simulink model "plt_aut_full"  (R2014a)
settings: Solver=ode45  StartTime=0.0  StopTime=70  MaxStep=0.01  RelTol=1e-3
values from neighbouring files (symbols this model uses):
  alpha = 1+1/(k*beta)    (= 1.025)    [tp1_syst_asservis.m]
  beta = 4    [tp1_syst_asservis.m]
  k = 10    [tp1_syst_asservis.m]
  Kd = 0.0001    [tp1_syst_asservis.m]
  Te = 0.2    [tp1_syst_asservis.m]
  to = 1.2    [tp1_syst_asservis.m]
settings Model: Creator=12210406  LastModifiedBy=UTILISATEUR
settings OptimizationCC: BlockReduction=off  BooleanDataType=off  SimCompilerOptimization=off
settings DebuggingCC: SaveWithParameterizedLinksMsg=none  UnderspecifiedInitializationDetection=Classic  SignalResolutionControl=TryResolveAllWithWarning  SolverPrmCheckMsg=none  FcnCallInpInsideContextMsg=error  FrameProcessingCompatibilityMsg=error  LibraryContextMissingDiagnostic=warning  SFExecutionAtInitializationDiag=none
settings HardwareCC: ProdBitPerSizeT=32  ProdBitPerPtrDiffT=32  TargetUnknown=on
settings RTWCC: RTWCompilerOptimization=off
settings CodeAppCC: StateflowObjectComments=on
settings ConfigComp: CovMetricSettings=dw  CovHtmlReporting=on  CovSaveCumulativeToWorkspaceVar=on  CovSaveSingleToWorkspaceVar=on  CovExternalEMLEnable=off  CovSFcnEnable=off

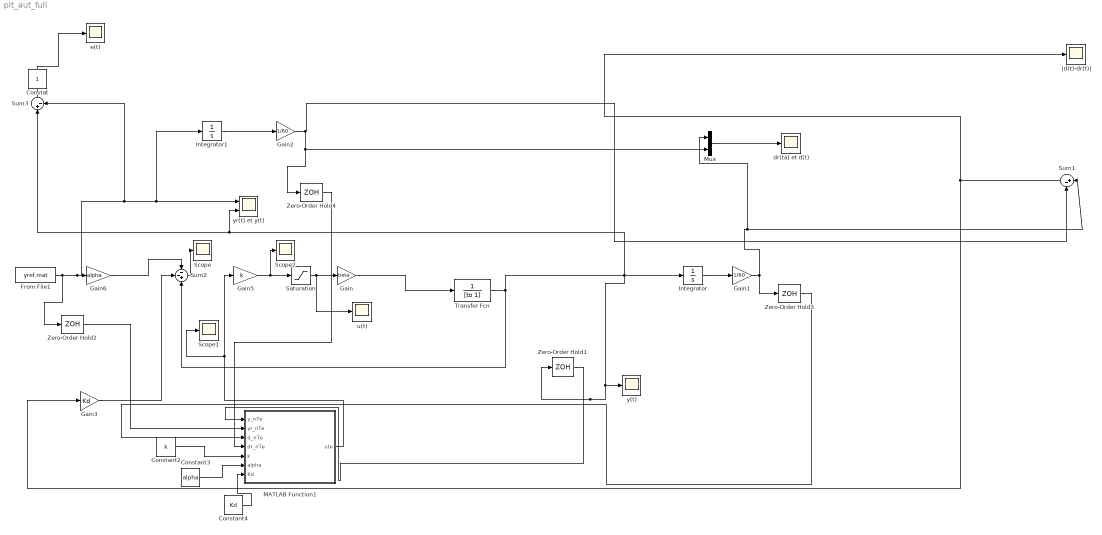
== system plt_aut_full ==
  Constant2 : Constant  Value=k
  Constant3 : Constant  Value=alpha
  Constant4 : Constant  Value=Kd
  From File1 : FromFile  FileName=yref.mat  SampleTime=0
  Gain : Gain  Gain=beta
  Gain1 : Gain  Gain=1/60
  Gain2 : Gain  Gain=1/60
  Gain3 : Gain  Gain=Kd
  Gain5 : Gain  Gain=k  ParamMax=[20]
  Gain6 : Gain  Gain=alpha
  Integrator : Integrator  UpperSaturationLimit=t  LowerSaturationLimit=0
  Integrator1 : Integrator  UpperSaturationLimit=t  LowerSaturationLimit=0
  MATLAB Function1 : MATLAB Function  TreatAsAtomicUnit=on
  Mux : Mux  Inputs=2
  Saturation : Saturate  UpperLimit=100  LowerLimit=-50
  Scope : Scope
      settings: SaveName=ScopeData3
  Scope1 : Scope
      settings: YMin=5000  YMax=13000  SaveName=ScopeData4
  Scope2 : Scope
      settings: YMin=-17500  YMax=7500  SaveName=ScopeData5
  Sum1 : Sum  Inputs=|+-
  Sum2 : Sum  Inputs=--+
  Sum3 : Sum  Inputs=|+-
  Transfer Fcn : TransferFcn  Denominator=[to 1]
  Zero-Order Hold{1..4} (4 alike) : ZeroOrderHold  SampleTime=Te
  dr(tà) et d(t) : Scope
  "e(t) " : Scope
  u(t) : Scope
      settings: TimeRange=50  YMin=-50  YMax=1000000  SaveName=ScopeData2  SampleInput=on
  y(t) : Scope
  yr(t) et y(t) : Scope  NumInputPorts=2
  "|d(t)-dr(t)| " : Scope
  Constat : Constant  IOType=siggen
  wires:
  Transfer Fcn/1 -> Sum2/3, Zero-Order Hold1/1, y(t)/1, yr(t) et y(t)/2, Sum3/1, Integrator/1
  Integrator/1 -> Gain1/1
  Saturation/1 -> u(t)/1, Gain/1
  Gain6/1 -> Sum2/1
  Gain5/1 -> Scope2/1, Saturation/1
  Integrator1/1 -> Gain2/1
  Gain2/1 -> Zero-Order Hold4/1, Mux/2, Sum1/2
  From File1/1 -> Zero-Order Hold2/1, Sum3/2, yr(t) et y(t)/1, Integrator1/1, Gain6/1
  Gain1/1 -> Mux/1, Sum1/1, Zero-Order Hold3/1
  Sum3/1 -> "e(t) "/1
  Sum1/1 -> "|d(t)-dr(t)| "/1, Gain3/1
  Gain3/1 -> Sum2/2
  Mux/1 -> dr(tà) et d(t)/1
  Zero-Order Hold1/1 -> MATLAB Function1/1(y_nTe)
  Zero-Order Hold2/1 -> MATLAB Function1/2(yr_nTe)
  Zero-Order Hold3/1 -> MATLAB Function1/3(d_nTe)
  Zero-Order Hold4/1 -> MATLAB Function1/4(dr_nTe)
  MATLAB Function1/1(ute) -> Gain5/1, Scope1/1
  Constant2/1 -> MATLAB Function1/5(k)
  Constant3/1 -> MATLAB Function1/6(alpha)
  Constant4/1 -> MATLAB Function1/7(Kd)
  Sum2/1 -> Scope/1
  Gain/1 -> Transfer Fcn/1

== matlab function plt_aut_full/MATLAB Function1 ==
  data: y_nTe input; ute output; yr_nTe input; d_nTe input; dr_nTe input; k input; alpha input; Kd input
function ute = fcn(y_nTe ,yr_nTe,d_nTe,dr_nTe,k,alpha,Kd)

%#codegen
ute= -k * (y_nTe-alpha*yr_nTe)-Kd*(d_nTe - dr_nTe);

end
